simulink model "Sys_CL"  (R2025b)
settings: Solver=VariableStepAuto  StartTime=0.0  StopTime=500  RelTol=1e-3
values from neighbouring files (symbols this model uses):
  C = [1, 0, 0]    [fase1.m]
  K = place(A, Bu, poles_SSF)    [fase1.m]
undefined symbols (not defined in the file or in its folder): ueq, xeq
settings Model: Creator=Rika  LastModifiedBy=Rika

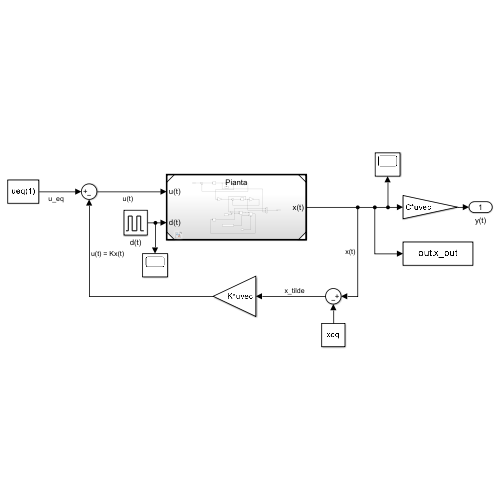
[thumbnail: Simulink's stored preview of the top-level diagram]
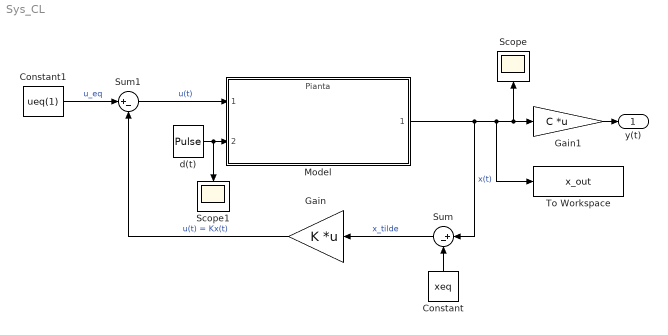
== system Sys_CL ==
  Constant : Constant  Value=xeq
  Constant1 : Constant  Value=ueq(1)
  Gain : Gain  Gain=K  Multiplication=Matrix(K*u) (u vector)
  Gain1 : Gain  Gain=C  Multiplication=Matrix(K*u) (u vector)
  Model : ModelReference  ModelNameDialog=Pianta.slx  SimulationMode=Normal  ModelReferenceVersion=1.16
  Scope : Scope
      settings: ActiveDisplayYMinimum=-171.91802446174057  ActiveDisplayYMaximum=420.64695014824434
  Scope1 : Scope
      settings: ActiveDisplayYMinimum=-31.975003621336949  ActiveDisplayYMaximum=2.8482216828598723
  Sum : Sum  Inputs=|+-
  Sum1 : Sum  Inputs=|+-
  To Workspace : ToWorkspace  VariableName=x_out  SampleTime=-1
  d(t) : DiscretePulseGenerator  PulseType=Time based  Amplitude=10  Period=1000  PulseWidth=3  PhaseDelay=10
  y(t) : Outport
  wires:
  Gain1/1 -> y(t)/1
  Sum/1 -> Gain/1  "x_tilde"
  Constant/1 -> Sum/2
  Constant1/1 -> Sum1/1  "u_eq"
  Sum1/1 -> Model/1  "u(t)"
  Gain/1 -> Sum1/2  "u(t) = Kx(t)"
  Model/1 -> To Workspace/1, Scope/1, Gain1/1, Sum/1  "x(t)"
  d(t)/1 -> Scope1/1, Model/2
